simulink model "MiniHelicopterControl"  (R2022b)
settings: Solver=FixedStepAuto  StartTime=0.0  StopTime=30  FixedStep=0.001  RelTol=1e-3
libraries: simulink x1
settings Model: PauseTimes=1  Creator=22438  LastModifiedBy=22438

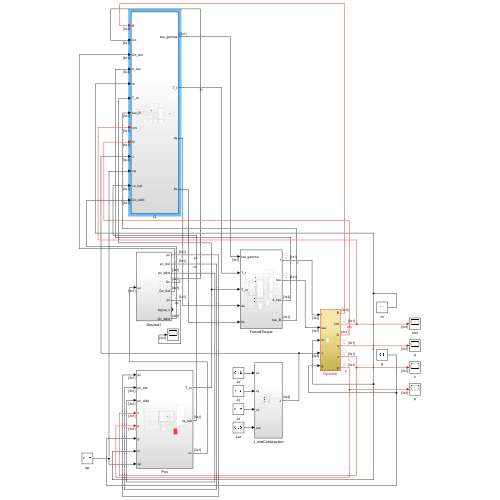
[thumbnail: Simulink's stored preview of the top-level diagram]
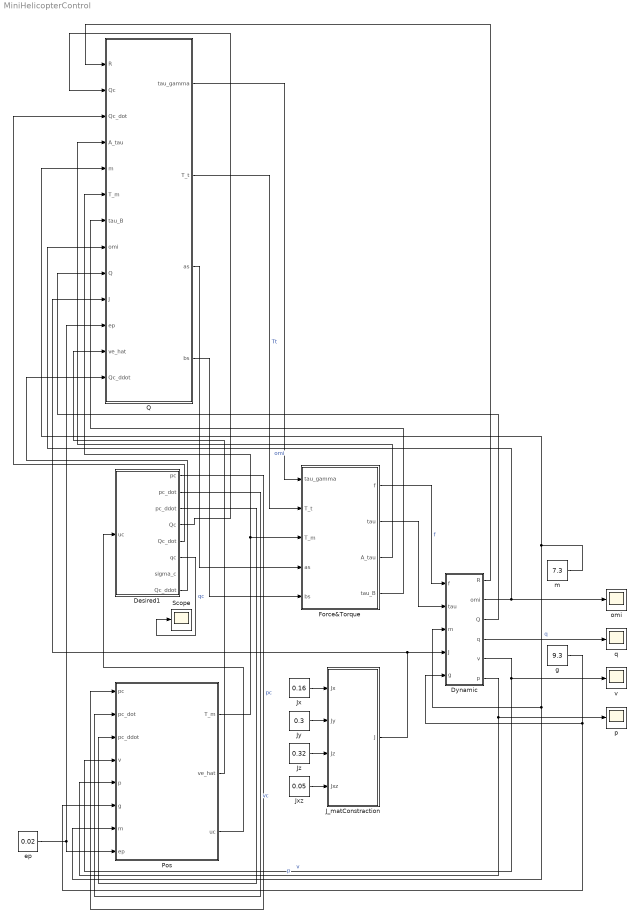
== system MiniHelicopterControl ==
  Desired1 : Subsystem
  Dynamic : Subsystem
  Force&Torque : Subsystem
  J_matConstraction : Subsystem
  Jx : Constant  Value=0.16
  Jxz : Constant  Value=0.05
  Jy : Constant  Value=0.3
  Jz : Constant  Value=0.32
  Pos : Subsystem
  Q : Subsystem
  Scope : Scope
  ep : Constant  Value=0.02
  g : Constant  Value=9.3
  m : Constant  Value=7.3
  omi : Scope
  p : Scope
  q : Scope
  v : Scope
  wires:
  J_matConstraction/1(J) -> Dynamic/4(J), Q/10(J)
  Desired1/1(pc) -> Pos/1(pc)  "pc"
  Desired1/2(pc_dot) -> Pos/2(pc_dot)  "vc"
  Desired1/3(pc_ddot) -> Pos/3(pc_ddot)
  Pos/1(T_m) -> Q/6(T_m), Force&Torque/3(T_m)
  Desired1/4(Qc) -> Q/2(Qc)
  Desired1/5(Qc_dot) -> Q/3(Qc_dot)
  Force&Torque/3(A_tau) -> Q/4(A_tau)
  Force&Torque/4(tau_B) -> Q/7(tau_B)
  ep/1 -> Pos/8(ep), Q/11(ep)
  Pos/2(ve_hat) -> Q/12(ve_hat)
  Q/1(tau_gamma) -> Force&Torque/1(tau_gamma)
  Q/2(T_t) -> Force&Torque/2(T_t)  "Tt"
  Jxz/1 -> J_matConstraction/4(Jxz)
  Jx/1 -> J_matConstraction/1(Jx)
  Jz/1 -> J_matConstraction/3(Jz)
  Jy/1 -> J_matConstraction/2(Jy)
  Q/3(as) -> Force&Torque/4(as)
  Q/4(bs) -> Force&Torque/5(bs)
  m/1 -> Q/5(m), Pos/7(m), Dynamic/3(m)
  Force&Torque/1(f) -> Dynamic/1(f)  "f"
  Force&Torque/2(tau) -> Dynamic/2(tau)
  Dynamic/1(R) -> Q/1(R)
  Dynamic/3(Q) -> Q/9(Q)
  Dynamic/4(q) -> q/1  "q"
  Dynamic/5(v) -> v/1, Pos/4(v)  "v"
  Dynamic/6(p) -> p/1, Pos/5(p)  "p"
  g/1 -> Dynamic/5(g), Pos/6(g)
  Dynamic/2(omi) -> omi/1, Q/8(omi)  "omi"
  Desired1/8(Qc_ddot) -> Q/13(Qc_ddot)
  Pos/3(uc) -> Desired1/1(uc)
  Desired1/6(qc) -> Scope/1  "qc"

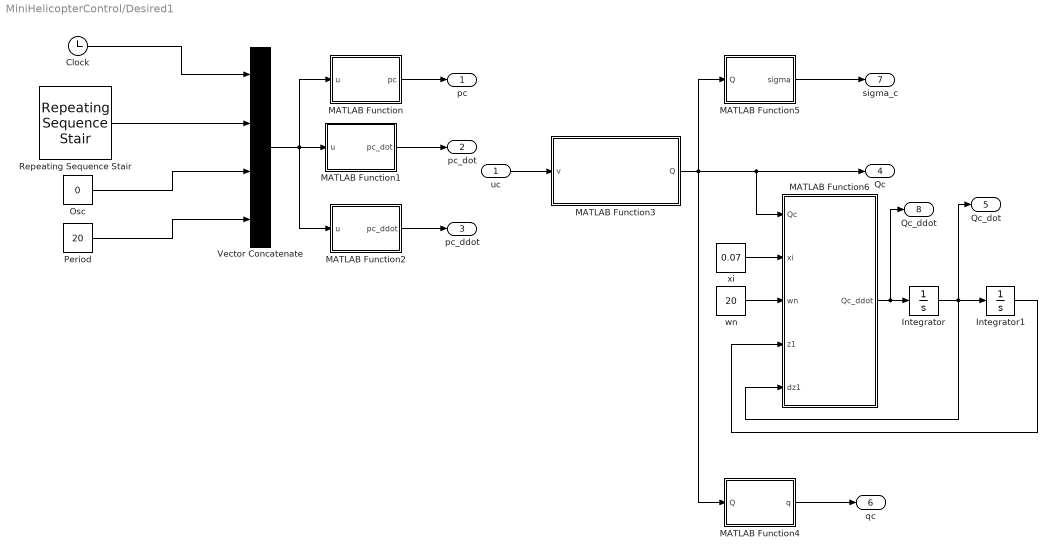
== system MiniHelicopterControl/Desired1 ==
  uc : Inport
  Clock : Clock
  Integrator : Integrator
  Integrator1 : Integrator
  MATLAB Function : MATLAB Function  TreatAsAtomicUnit=on
  MATLAB Function1 : MATLAB Function  TreatAsAtomicUnit=on
  MATLAB Function2 : MATLAB Function  TreatAsAtomicUnit=on
  MATLAB Function3 : MATLAB Function  TreatAsAtomicUnit=on
  MATLAB Function4 : MATLAB Function  TreatAsAtomicUnit=on
  MATLAB Function5 : MATLAB Function  TreatAsAtomicUnit=on
  MATLAB Function6 : MATLAB Function  TreatAsAtomicUnit=on
  Osc : Constant  Value=0
  Period : Constant  Value=20
  Repeating Sequence Stair : simulink/Sources/Repeating Sequence Stair  OutValues=[3].'  tsamp=-1  OutMin=[]  OutMax=[]  OutDataTypeStr=double  OutputDataTypeScalingMode=double  OutDataType=fixdt(0,8)  ConRadixGroup=Best Precision: Vector-wise  OutScaling=2^-12
  Vector Concatenate : Concatenate  NumInputs=4
  wn : Constant  Value=20
  xi : Constant  Value=0.07
  pc : Outport
  pc_dot : Outport  Port=2
  pc_ddot : Outport  Port=3
  Qc : Outport  Port=4
  Qc_dot : Outport  Port=5
  qc : Outport  Port=6
  sigma_c : Outport  Port=7
  Qc_ddot : Outport  Port=8
  wires:
  Repeating Sequence Stair/1 -> Vector Concatenate/2
  Period/1 -> Vector Concatenate/4
  Clock/1 -> Vector Concatenate/1
  MATLAB Function/1(pc) -> pc/1
  Osc/1 -> Vector Concatenate/3
  Vector Concatenate/1 -> MATLAB Function2/1(u), MATLAB Function1/1(u), MATLAB Function/1(u)
  MATLAB Function1/1(pc_dot) -> pc_dot/1
  MATLAB Function2/1(pc_ddot) -> pc_ddot/1
  MATLAB Function4/1(q) -> qc/1
  MATLAB Function5/1(sigma) -> sigma_c/1
  MATLAB Function3/1(Q) -> MATLAB Function4/1(Q), MATLAB Function5/1(Q), Qc/1, MATLAB Function6/1(Qc)
  xi/1 -> MATLAB Function6/2(xi)
  wn/1 -> MATLAB Function6/3(wn)
  MATLAB Function6/1(Qc_ddot) -> Qc_ddot/1, Integrator/1
  Integrator/1 -> Qc_dot/1, MATLAB Function6/5(dz1), Integrator1/1
  Integrator1/1 -> MATLAB Function6/4(z1)
  uc/1 -> MATLAB Function3/1(v)

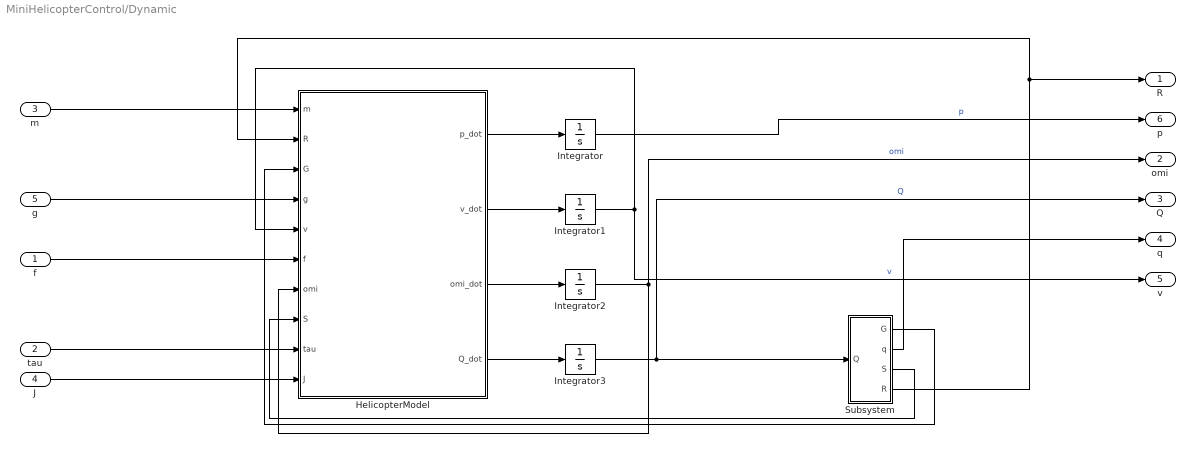
== system MiniHelicopterControl/Dynamic ==
  f : Inport
  tau : Inport  Port=2
  m : Inport  Port=3
  J : Inport  Port=4
  g : Inport  Port=5
  HelicopterModel : MATLAB Function  TreatAsAtomicUnit=on
  Integrator : Integrator  InitialCondition=[1;1;0]
  Integrator1 : Integrator
  Integrator2 : Integrator
  Integrator3 : Integrator  InitialCondition=[sqrt(3)/2;1/2;0;0]
  Subsystem : Subsystem
  R : Outport
  omi : Outport  Port=2
  Q : Outport  Port=3
  q : Outport  Port=4
  v : Outport  Port=5
  p : Outport  Port=6
  wires:
  Integrator1/1 -> v/1, HelicopterModel/5(v)  "v"
  Integrator3/1 -> Subsystem/1(Q), Q/1  "Q"
  Integrator2/1 -> omi/1, HelicopterModel/7(omi)  "omi"
  HelicopterModel/4(Q_dot) -> Integrator3/1
  Integrator/1 -> p/1  "p"
  HelicopterModel/3(omi_dot) -> Integrator2/1
  HelicopterModel/1(p_dot) -> Integrator/1
  J/1 -> HelicopterModel/10(J)
  HelicopterModel/2(v_dot) -> Integrator1/1
  g/1 -> HelicopterModel/4(g)
  tau/1 -> HelicopterModel/9(tau)
  f/1 -> HelicopterModel/6(f)
  m/1 -> HelicopterModel/1(m)
  Subsystem/4(R) -> HelicopterModel/2(R), R/1
  Subsystem/1(G) -> HelicopterModel/3(G)
  Subsystem/2(q) -> q/1
  Subsystem/3(S) -> HelicopterModel/8(S)

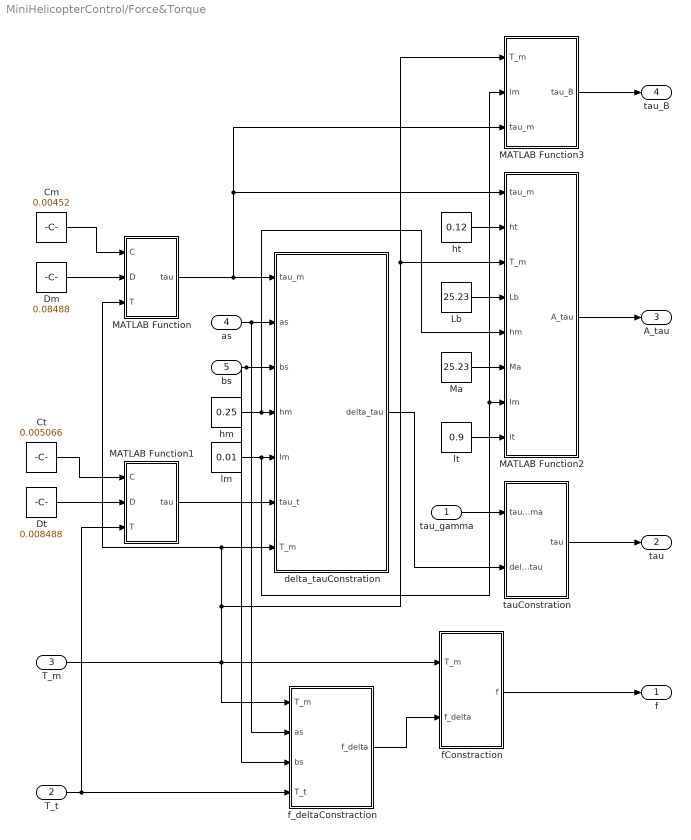
== system MiniHelicopterControl/Force&Torque ==
  tau_gamma : Inport
  T_t : Inport  Port=2
  T_m : Inport  Port=3
  as : Inport  Port=4
  bs : Inport  Port=5
  Cm : Constant  Value=0.00452
  Ct : Constant  Value=0.005066
  Dm : Constant  Value=0.08488
  Dt : Constant  Value=0.008488
  Lb : Constant  Value=25.23
  MATLAB Function : MATLAB Function  TreatAsAtomicUnit=on
  MATLAB Function1 : MATLAB Function  TreatAsAtomicUnit=on
  MATLAB Function2 : MATLAB Function  TreatAsAtomicUnit=on
  MATLAB Function3 : MATLAB Function  TreatAsAtomicUnit=on
  Ma : Constant  Value=25.23
  delta_tauConstration : MATLAB Function  TreatAsAtomicUnit=on
  fConstraction : MATLAB Function  TreatAsAtomicUnit=on
  f_deltaConstraction : MATLAB Function  TreatAsAtomicUnit=on
  hm : Constant  Value=0.25
  ht : Constant  Value=0.12
  lm : Constant  Value=0.01
  lt : Constant  Value=0.9
  tauConstration : MATLAB Function  TreatAsAtomicUnit=on
  f : Outport
  tau : Outport  Port=2
  A_tau : Outport  Port=3
  tau_B : Outport  Port=4
  wires:
  as/1 -> f_deltaConstraction/2(as), delta_tauConstration/2(as)
  delta_tauConstration/1(delta_tau) -> tauConstration/2(delta_tau)
  lm/1 -> MATLAB Function3/2(lm), MATLAB Function2/7(lm), delta_tauConstration/5(lm)
  T_m/1 -> f_deltaConstraction/1(T_m), fConstraction/1(T_m), MATLAB Function3/1(T_m), MATLAB Function2/3(T_m), MATLAB Function/3(T), delta_tauConstration/7(T_m)
  bs/1 -> delta_tauConstration/3(bs), f_deltaConstraction/3(bs)
  f_deltaConstraction/1(f_delta) -> fConstraction/2(f_delta)
  hm/1 -> MATLAB Function2/5(hm), delta_tauConstration/4(hm)
  T_t/1 -> MATLAB Function1/3(T), f_deltaConstraction/4(T_t)
  MATLAB Function1/1(tau) -> delta_tauConstration/6(tau_t)
  tau_gamma/1 -> tauConstration/1(tau_gamma)
  fConstraction/1(f) -> f/1
  tauConstration/1(tau) -> tau/1
  MATLAB Function/1(tau) -> MATLAB Function3/3(tau_m), MATLAB Function2/1(tau_m), delta_tauConstration/1(tau_m)
  Cm/1 -> MATLAB Function/1(C)
  Dm/1 -> MATLAB Function/2(D)
  Ct/1 -> MATLAB Function1/1(C)
  Dt/1 -> MATLAB Function1/2(D)
  ht/1 -> MATLAB Function2/2(ht)
  Lb/1 -> MATLAB Function2/4(Lb)
  Ma/1 -> MATLAB Function2/6(Ma)
  lt/1 -> MATLAB Function2/8(lt)
  MATLAB Function2/1(A_tau) -> A_tau/1
  MATLAB Function3/1(tau_B) -> tau_B/1

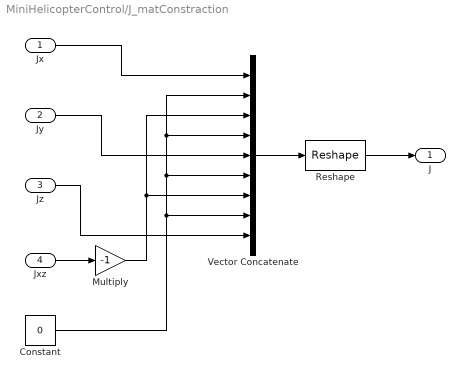
== system MiniHelicopterControl/J_matConstraction ==
  Jx : Inport
  Jy : Inport  Port=2
  Jz : Inport  Port=3
  Jxz : Inport  Port=4
  Constant : Constant  Value=0
  Multiply : Gain  Gain=-1
  Reshape : Reshape  OutputDimensionality=Customize  OutputDimensions=[3,3]
  Vector Concatenate : Concatenate  NumInputs=9
  J : Outport
  wires:
  Jy/1 -> Vector Concatenate/5
  Vector Concatenate/1 -> Reshape/1
  Constant/1 -> Vector Concatenate/8, Vector Concatenate/6, Vector Concatenate/4, Vector Concatenate/2
  Jz/1 -> Vector Concatenate/9
  Jx/1 -> Vector Concatenate/1
  Reshape/1 -> J/1
  Multiply/1 -> Vector Concatenate/7, Vector Concatenate/3
  Jxz/1 -> Multiply/1

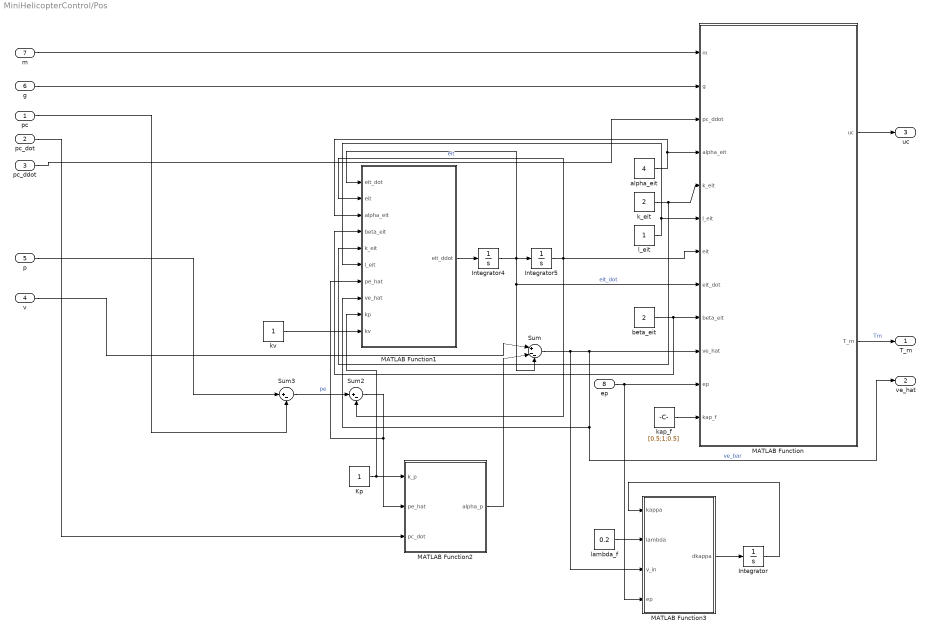
== system MiniHelicopterControl/Pos ==
  pc : Inport
  pc_dot : Inport  Port=2
  pc_ddot : Inport  Port=3
  v : Inport  Port=4
  p : Inport  Port=5
  g : Inport  Port=6
  m : Inport  Port=7
  ep : Inport  Port=8
  Integrator : Integrator
  Integrator4 : Integrator
  Integrator5 : Integrator  InitialCondition=[0.3;0.3;0.3]
  Kp : Constant
  MATLAB Function : MATLAB Function  TreatAsAtomicUnit=on
  MATLAB Function1 : MATLAB Function  TreatAsAtomicUnit=on
  MATLAB Function2 : MATLAB Function  TreatAsAtomicUnit=on
  MATLAB Function3 : MATLAB Function  TreatAsAtomicUnit=on
  Sum : Sum  Inputs=|+--
  Sum2 : Sum  Inputs=|+-
  Sum3 : Sum  Inputs=|+-
  alpha_eit : Constant  Value=4
  beta_eit : Constant  Value=2
  k_eit : Constant  Value=2
  kap_f : Constant  Value=[0.5;1;0.5]
  kv : Constant
  l_eit : Constant
  lambda_f : Constant  Value=0.2
  T_m : Outport
  ve_hat : Outport  Port=2
  uc : Outport  Port=3
  wires:
  k_eit/1 -> MATLAB Function1/5(k_eit), MATLAB Function/5(k_eit)
  beta_eit/1 -> MATLAB Function1/4(beta_eit), MATLAB Function/9(beta_eit)
  Integrator5/1 -> Sum2/2, MATLAB Function/7(eit), MATLAB Function1/2(eit)  "eit"
  l_eit/1 -> MATLAB Function1/6(l_eit), MATLAB Function/6(l_eit)
  Integrator4/1 -> Integrator5/1, MATLAB Function/8(eit_dot), Sum/3, MATLAB Function1/1(eit_dot)  "eit_dot"
  Sum2/1 -> MATLAB Function1/7(pe_hat), MATLAB Function2/2(pe_hat)
  alpha_eit/1 -> MATLAB Function1/3(alpha_eit), MATLAB Function/4(alpha_eit)
  MATLAB Function/2(T_m) -> T_m/1  "Tm"
  MATLAB Function1/1(eit_ddot) -> Integrator4/1
  Integrator/1 -> MATLAB Function3/1(kappa)
  MATLAB Function2/1(alpha_p) -> Sum/2
  v/1 -> Sum/1
  ep/1 -> MATLAB Function3/4(ep), MATLAB Function/11(ep)
  p/1 -> Sum3/1
  Sum3/1 -> Sum2/1  "pe"
  pc_dot/1 -> MATLAB Function2/3(pc_dot)
  pc_ddot/1 -> MATLAB Function/3(pc_ddot)
  pc/1 -> Sum3/2
  g/1 -> MATLAB Function/2(g)
  m/1 -> MATLAB Function/1(m)
  Kp/1 -> MATLAB Function1/9(kp), MATLAB Function2/1(k_p)
  kv/1 -> MATLAB Function1/10(kv)
  MATLAB Function/1(uc) -> uc/1
  MATLAB Function3/1(dkappa) -> Integrator/1
  lambda_f/1 -> MATLAB Function3/2(lambda)
  Sum/1 -> MATLAB Function3/3(v_in), MATLAB Function1/8(ve_hat), ve_hat/1, MATLAB Function/10(ve_hat)  "ve_bar"
  kap_f/1 -> MATLAB Function/12(kap_f)

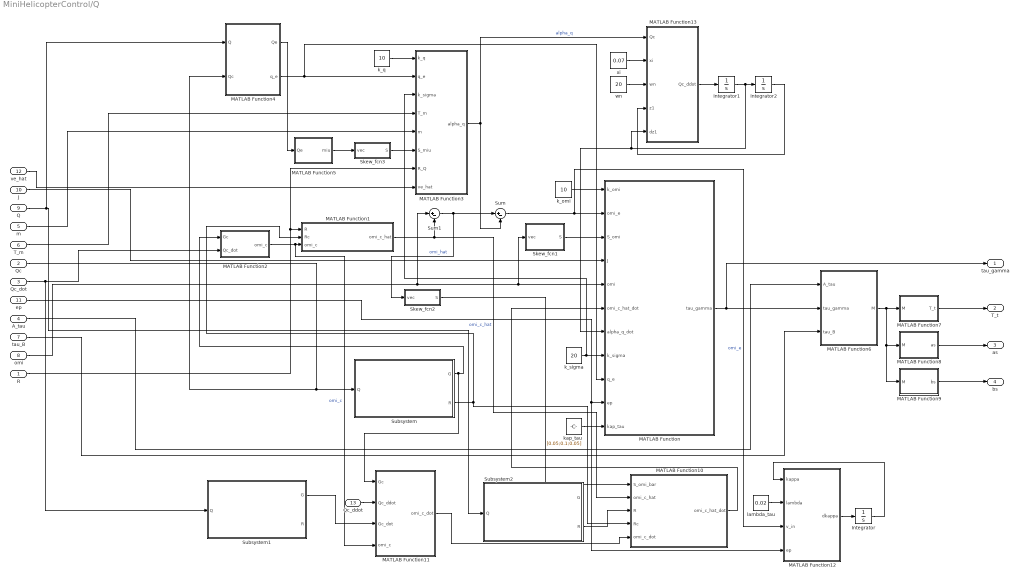
== system MiniHelicopterControl/Q ==
  R : Inport
  Qc : Inport  Port=2
  Qc_dot : Inport  Port=3
  A_tau : Inport  Port=4
  m : Inport  Port=5
  T_m : Inport  Port=6
  tau_B : Inport  Port=7
  omi : Inport  Port=8
  Q : Inport  Port=9
  J : Inport  Port=10
  ep : Inport  Port=11
  ve_hat : Inport  Port=12
  Qc_ddot : Inport  Port=13
  Integrator : Integrator
  Integrator1 : Integrator
  Integrator2 : Integrator
  MATLAB Function : MATLAB Function  TreatAsAtomicUnit=on
  MATLAB Function1 : MATLAB Function  TreatAsAtomicUnit=on
  MATLAB Function10 : MATLAB Function  TreatAsAtomicUnit=on
  MATLAB Function11 : MATLAB Function  TreatAsAtomicUnit=on
  MATLAB Function12 : MATLAB Function  TreatAsAtomicUnit=on
  MATLAB Function13 : MATLAB Function  TreatAsAtomicUnit=on
  MATLAB Function2 : MATLAB Function  TreatAsAtomicUnit=on
  MATLAB Function3 : MATLAB Function  TreatAsAtomicUnit=on
  MATLAB Function4 : MATLAB Function  TreatAsAtomicUnit=on
  MATLAB Function5 : MATLAB Function  TreatAsAtomicUnit=on
  MATLAB Function6 : MATLAB Function  TreatAsAtomicUnit=on
  MATLAB Function7 : MATLAB Function  TreatAsAtomicUnit=on
  MATLAB Function8 : MATLAB Function  TreatAsAtomicUnit=on
  MATLAB Function9 : MATLAB Function  TreatAsAtomicUnit=on
  Skew_fcn1 : MATLAB Function  TreatAsAtomicUnit=on
  Skew_fcn2 : MATLAB Function  TreatAsAtomicUnit=on
  Skew_fcn3 : MATLAB Function  TreatAsAtomicUnit=on
  Subsystem : Subsystem
  Subsystem1 : Subsystem
  Subsystem2 : Subsystem
  Sum : Sum  Inputs=|+-
  Sum1 : Sum  Inputs=|+-
  k_omi : Constant  Value=10
  k_q : Constant  Value=10
  k_sigma : Constant  Value=20
  kap_tau : Constant  Value=[0.05;0.1;0.05]
  lambda_tau : Constant  Value=0.02
  wn : Constant  Value=20
  xi : Constant  Value=0.07
  tau_gamma : Outport
  T_t : Outport  Port=2
  as : Outport  Port=3
  bs : Outport  Port=4
  wires:
  T_m/1 -> MATLAB Function3/4(T_m)
  A_tau/1 -> MATLAB Function6/1(A_tau)
  Integrator/1 -> MATLAB Function12/1(kappa)
  MATLAB Function3/1(alpha_q) -> MATLAB Function13/1(Qc), Sum/2  "alpha_q"
  MATLAB Function/1(tau_gamma) -> tau_gamma/1, MATLAB Function6/2(tau_gamma)
  k_q/1 -> MATLAB Function3/1(k_q)
  k_sigma/1 -> MATLAB Function3/3(k_sigma), MATLAB Function/8(k_sigma)
  Qc/1 -> Subsystem/1(Q), MATLAB Function4/2(Qc)
  MATLAB Function4/2(q_e) -> MATLAB Function/9(q_e), MATLAB Function3/2(q_e)
  ep/1 -> MATLAB Function12/4(ep), MATLAB Function/10(ep)
  Q/1 -> Subsystem2/1(Q), MATLAB Function4/1(Q)
  omi/1 -> Skew_fcn1/1(vec), MATLAB Function/5(omi), Sum1/1
  MATLAB Function6/1(M) -> MATLAB Function9/1(M), MATLAB Function8/1(M), MATLAB Function7/1(M)
  MATLAB Function1/1(omi_c_hat) -> MATLAB Function10/2(omi_c_hat), Sum1/2  "omi_c_hat"
  MATLAB Function4/1(Qe) -> MATLAB Function5/1(Qe)
  Sum/1 -> MATLAB Function12/3(v_in), MATLAB Function/2(omi_e)  "omi_e"
  Skew_fcn1/1(S) -> MATLAB Function/3(S_omi)
  Integrator1/1 -> MATLAB Function/7(alpha_q_dot), MATLAB Function13/5(dz1), Integrator2/1
  Sum1/1 -> Skew_fcn2/1(vec), Sum/1  "omi_hat"
  ve_hat/1 -> MATLAB Function3/8(ve_hat)
  MATLAB Function5/1(miu) -> Skew_fcn3/1(vec)
  Skew_fcn3/1(S) -> MATLAB Function3/6(S_miu)
  R/1 -> MATLAB Function3/7(R_Q), MATLAB Function1/1(R)
  MATLAB Function2/1(omi_c) -> MATLAB Function11/4(omi_c), MATLAB Function1/3(omi_c)  "omi_c"
  J/1 -> MATLAB Function/4(J)
  k_omi/1 -> MATLAB Function/1(k_omi)
  m/1 -> MATLAB Function3/5(m)
  Qc_dot/1 -> Subsystem1/1(Q), MATLAB Function2/2(Qc_dot)
  tau_B/1 -> MATLAB Function6/3(tau_B)
  MATLAB Function7/1(T_t) -> T_t/1
  MATLAB Function8/1(as) -> as/1
  MATLAB Function9/1(bs) -> bs/1
  Subsystem/1(G) -> MATLAB Function11/1(Gc), MATLAB Function2/1(Gc)
  Subsystem/2(R) -> MATLAB Function1/2(Rc), MATLAB Function10/4(Rc)
  MATLAB Function10/1(omi_c_hat_dot) -> MATLAB Function/6(omi_c_hat_dot)
  Skew_fcn2/1(S) -> MATLAB Function10/1(S_omi_bar)
  Subsystem1/1(G) -> MATLAB Function11/3(Gc_dot)
  Qc_ddot/1 -> MATLAB Function11/2(Qc_ddot)
  MATLAB Function11/1(omi_c_dot) -> MATLAB Function10/5(omi_c_dot)
  Subsystem2/2(R) -> MATLAB Function10/3(R)
  MATLAB Function12/1(dkappa) -> Integrator/1
  lambda_tau/1 -> MATLAB Function12/2(lambda)
  kap_tau/1 -> MATLAB Function/11(kap_tau)
  xi/1 -> MATLAB Function13/2(xi)
  wn/1 -> MATLAB Function13/3(wn)
  MATLAB Function13/1(Qc_ddot) -> Integrator1/1
  Integrator2/1 -> MATLAB Function13/4(z1)

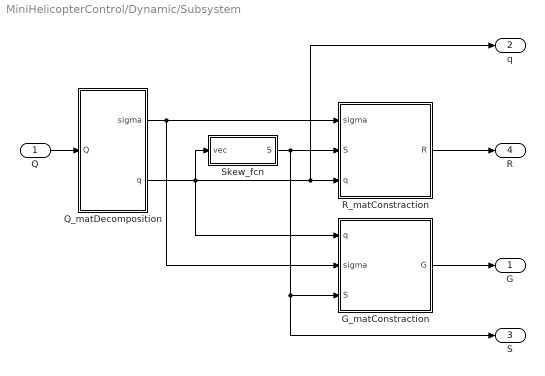
== system MiniHelicopterControl/Dynamic/Subsystem ==
  Q : Inport
  G_matConstraction : MATLAB Function  TreatAsAtomicUnit=on
  Q_matDecomposition : MATLAB Function  TreatAsAtomicUnit=on
  R_matConstraction : MATLAB Function  TreatAsAtomicUnit=on
  Skew_fcn : MATLAB Function  TreatAsAtomicUnit=on
  G : Outport
  q : Outport  Port=2
  S : Outport  Port=3
  R : Outport  Port=4
  wires:
  Q/1 -> Q_matDecomposition/1(Q)
  Q_matDecomposition/2(q) -> Skew_fcn/1(vec), q/1, R_matConstraction/3(q), G_matConstraction/1(q)
  R_matConstraction/1(R) -> R/1
  Skew_fcn/1(S) -> S/1, G_matConstraction/3(S), R_matConstraction/2(S)
  Q_matDecomposition/1(sigma) -> G_matConstraction/2(sigma), R_matConstraction/1(sigma)
  G_matConstraction/1(G) -> G/1

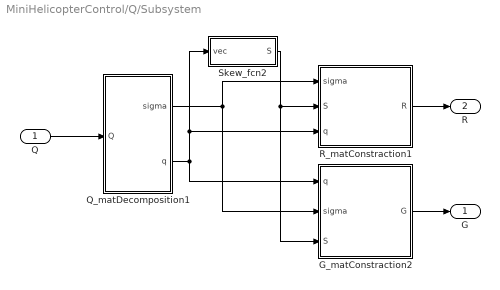
== system MiniHelicopterControl/Q/Subsystem ==
  Q : Inport
  G_matConstraction2 : MATLAB Function  TreatAsAtomicUnit=on
  Q_matDecomposition1 : MATLAB Function  TreatAsAtomicUnit=on
  R_matConstraction1 : MATLAB Function  TreatAsAtomicUnit=on
  Skew_fcn2 : MATLAB Function  TreatAsAtomicUnit=on
  G : Outport
  R : Outport  Port=2
  wires:
  Q_matDecomposition1/2(q) -> Skew_fcn2/1(vec), R_matConstraction1/3(q), G_matConstraction2/1(q)
  R_matConstraction1/1(R) -> R/1
  Skew_fcn2/1(S) -> G_matConstraction2/3(S), R_matConstraction1/2(S)
  Q_matDecomposition1/1(sigma) -> R_matConstraction1/1(sigma), G_matConstraction2/2(sigma)
  G_matConstraction2/1(G) -> G/1
  Q/1 -> Q_matDecomposition1/1(Q)

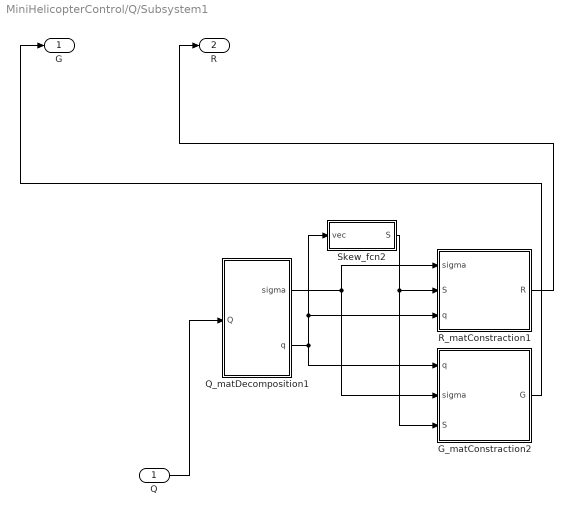
== system MiniHelicopterControl/Q/Subsystem1 ==
  Q : Inport
  G_matConstraction2 : MATLAB Function  TreatAsAtomicUnit=on
  Q_matDecomposition1 : MATLAB Function  TreatAsAtomicUnit=on
  R_matConstraction1 : MATLAB Function  TreatAsAtomicUnit=on
  Skew_fcn2 : MATLAB Function  TreatAsAtomicUnit=on
  G : Outport
  R : Outport  Port=2
  wires:
  Q_matDecomposition1/2(q) -> Skew_fcn2/1(vec), R_matConstraction1/3(q), G_matConstraction2/1(q)
  R_matConstraction1/1(R) -> R/1
  Skew_fcn2/1(S) -> G_matConstraction2/3(S), R_matConstraction1/2(S)
  Q_matDecomposition1/1(sigma) -> R_matConstraction1/1(sigma), G_matConstraction2/2(sigma)
  G_matConstraction2/1(G) -> G/1
  Q/1 -> Q_matDecomposition1/1(Q)

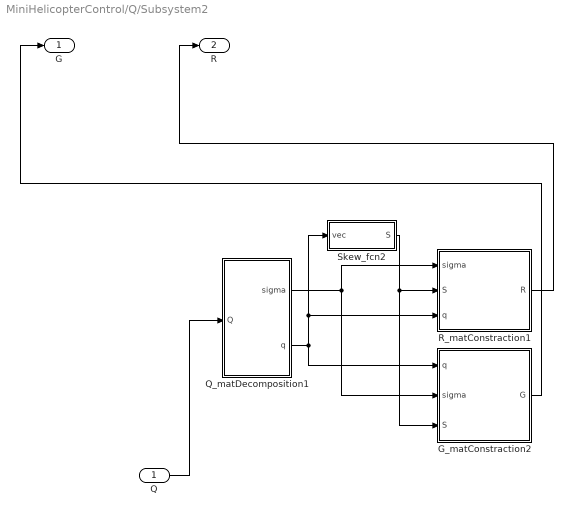
== system MiniHelicopterControl/Q/Subsystem2 ==
  Q : Inport
  G_matConstraction2 : MATLAB Function  TreatAsAtomicUnit=on
  Q_matDecomposition1 : MATLAB Function  TreatAsAtomicUnit=on
  R_matConstraction1 : MATLAB Function  TreatAsAtomicUnit=on
  Skew_fcn2 : MATLAB Function  TreatAsAtomicUnit=on
  G : Outport
  R : Outport  Port=2
  wires:
  Q_matDecomposition1/2(q) -> Skew_fcn2/1(vec), R_matConstraction1/3(q), G_matConstraction2/1(q)
  R_matConstraction1/1(R) -> R/1
  Skew_fcn2/1(S) -> G_matConstraction2/3(S), R_matConstraction1/2(S)
  Q_matDecomposition1/1(sigma) -> R_matConstraction1/1(sigma), G_matConstraction2/2(sigma)
  G_matConstraction2/1(G) -> G/1
  Q/1 -> Q_matDecomposition1/1(Q)

== matlab function MiniHelicopterControl/Q/MATLAB Function10 ==
  data: omi_c_hat_dot output; S_omi_bar input; omi_c_hat input; R input; Rc input; omi_c_dot input
function omi_c_hat_dot = fcn(S_omi_bar, omi_c_hat, R, Rc, omi_c_dot)
omi_c_hat_dot = -S_omi_bar*omi_c_hat + R*Rc'*omi_c_dot;
end

== matlab function MiniHelicopterControl/Q/Skew_fcn2 ==
  data: vec input; S output
function S = fcn(vec)
v = vec;
vx = v(1);
vy = v(2);
vz = v(3);

S = [ ...
    0, -vz, vy; ...
    vz, 0, -vx; ...
    -vy, vx, 0 ...
    ];
end

== matlab function MiniHelicopterControl/Q/MATLAB Function11 ==
  data: Gc input; omi_c_dot output; Qc_ddot input; Gc_dot input; omi_c input
function omi_c_dot = fcn(Gc, Qc_ddot, Gc_dot, omi_c)
omi_c_dot = Gc'*(Qc_ddot - Gc_dot*omi_c);
end

== matlab function MiniHelicopterControl/Pos/MATLAB Function ==
  data: uc output size=[3 1]; m input; g input; T_m output size=1; pc_ddot input; alpha_eit input; k_eit input; l_eit input; eit input; eit_dot input; beta_eit input; ve_hat input; ep input; kap_f input
function [uc,T_m]= fcn(m, g, pc_ddot, alpha_eit, k_eit, l_eit, eit, eit_dot, beta_eit, ve_hat, ep, kap_f)
uc = g.*[0;0;1] + pc_ddot - alpha_eit.*tanh(k_eit.*eit + l_eit.*eit_dot) - ...
    beta_eit.*tanh(l_eit.*eit_dot) - tanh(diag(ve_hat./ep))*kap_f;
T_m = m*norm(uc);
end

== matlab function MiniHelicopterControl/Pos/MATLAB Function3 ==
  data: kappa input; dkappa output; lambda input; v_in input; ep input
function dkappa = fcn(kappa, lambda, v_in, ep)
dkappa = lambda*tanh(v_in/ep).*v_in-0.002*kappa;
end

== matlab function MiniHelicopterControl/Q/Subsystem1/G_matConstraction2 ==
  data: q input; sigma input; G output; S input
function G = fcn(q, sigma, S)
G = 0.5.*[-1.*q';...
    sigma.*eye(3) + S];
end

== matlab function MiniHelicopterControl/Q/Subsystem1/Q_matDecomposition1 ==
  data: Q input; sigma output; q output
function [sigma, q] = fcn(Q)
sigma = Q(1);
q = [Q(2);Q(3);Q(4)];
end

== matlab function MiniHelicopterControl/Q/MATLAB Function12 ==
  data: kappa input; dkappa output; lambda input; v_in input; ep input
function dkappa = fcn(kappa, lambda, v_in, ep)
dkappa = lambda*tanh(v_in/ep).*v_in-0.002*kappa;
end

== matlab function MiniHelicopterControl/Q/Subsystem1/R_matConstraction1 ==
  data: sigma input; R output; S input; q input
function R = fcn(sigma, S, q)
R = (sigma^2 - q'*q)*eye(3) + 2*q*q' - 2*sigma*S;
end

== matlab function MiniHelicopterControl/Dynamic/Subsystem/Q_matDecomposition ==
  data: Q input; sigma output; q output
function [sigma, q] = fcn(Q)
sigma = Q(1);
q = [Q(2);Q(3);Q(4)];
end

== matlab function MiniHelicopterControl/Pos/MATLAB Function1 ==
  data: eit_dot input; eit_ddot output; eit input; alpha_eit input; beta_eit input; k_eit input; l_eit input; pe_hat input; ve_hat input; kp input; kv input
function eit_ddot = fcn(eit_dot, eit, alpha_eit, beta_eit, k_eit, l_eit, pe_hat, ve_hat, kp, kv)
eit_ddot = -alpha_eit.*tanh(k_eit.*eit + l_eit.*eit_dot) - beta_eit.*tanh(l_eit.*eit_dot) - (kp^2-1)*pe_hat + (kv+kp)*ve_hat;
end

== matlab function MiniHelicopterControl/Pos/MATLAB Function2 ==
  data: k_p input; alpha_p output; pe_hat input; pc_dot input
function alpha_p = fcn(k_p, pe_hat, pc_dot)
alpha_p = -k_p.*pe_hat + pc_dot;
end

== matlab function MiniHelicopterControl/Force&Torque/MATLAB Function ==
  data: C input; tau output; D input; T input
function tau = fcn(C, D, T)
tau = C*abs(T)^1.5 + D;
end

== matlab function MiniHelicopterControl/Force&Torque/MATLAB Function1 ==
  data: C input; tau output; D input; T input
function tau = fcn(C, D, T)
tau = C*abs(T)^1.5 + D;
end

== matlab function MiniHelicopterControl/Q/MATLAB Function ==
  data: k_omi input; tau_gamma output size=[3 1]; omi_e input; S_omi input; J input; omi input; omi_c_hat_dot input; alpha_q_dot input; k_sigma input; q_e input; ep input; kap_tau input
function tau_gamma = fcn(k_omi, omi_e, S_omi, J, omi, omi_c_hat_dot, alpha_q_dot, k_sigma, q_e, ep, kap_tau)
tau_gamma = -k_omi*omi_e + S_omi*J*omi + J*(omi_c_hat_dot+alpha_q_dot) - k_sigma*q_e - tanh(diag(omi_e./ep))*kap_tau;
end

== matlab function MiniHelicopterControl/Q/Skew_fcn1 ==
  data: vec input; S output
function S = fcn(vec)
v = vec;
vx = v(1);
vy = v(2);
vz = v(3);

S = [ ...
    0, -vz, vy; ...
    vz, 0, -vx; ...
    -vy, vx, 0 ...
    ];
end

== matlab function MiniHelicopterControl/Q/MATLAB Function1 ==
  data: R input; omi_c_hat output; Rc input; omi_c input
function omi_c_hat = fcn(R, Rc, omi_c)
omi_c_hat = R*Rc'*omi_c;
end

== matlab function MiniHelicopterControl/Dynamic/HelicopterModel ==
  data: m input; p_dot output size=[3 1]; R input; G input; g input; v input; f input; omi input; S input; tau input; J input; v_dot output size=[3 1]; omi_dot output size=[3 1]; Q_dot output size=[4 1]
function [p_dot, v_dot, omi_dot, Q_dot] = fcn(m, R, G, g, v, f, omi, S, tau, J)
p_dot = v;
v_dot = -g.*[0; 0; 1] + 1/m*R'*f;
Q_dot = G*omi;
omi_dot = J^(-1)*(-1*S*J*omi + tau);
end

== matlab function MiniHelicopterControl/Q/Subsystem/Q_matDecomposition1 ==
  data: Q input; sigma output; q output
function [sigma, q] = fcn(Q)
sigma = Q(1);
q = [Q(2);Q(3);Q(4)];
end

== matlab function MiniHelicopterControl/Q/Subsystem/R_matConstraction1 ==
  data: sigma input; R output; S input; q input
function R = fcn(sigma, S, q)
R = (sigma^2 - q'*q)*eye(3) + 2*(q*q') - 2*sigma*S;
end

== matlab function MiniHelicopterControl/Q/Subsystem/Skew_fcn2 ==
  data: vec input; S output
function S = fcn(vec)
v = vec;
vx = v(1);
vy = v(2);
vz = v(3);

S = [ ...
    0, -vz, vy; ...
    vz, 0, -vx; ...
    -vy, vx, 0 ...
    ];
end

== matlab function MiniHelicopterControl/Q/Skew_fcn3 ==
  data: vec input; S output
function S = fcn(vec)
v = vec;
vx = v(1);
vy = v(2);
vz = v(3);

S = [ ...
    0, -vz, vy; ...
    vz, 0, -vx; ...
    -vy, vx, 0 ...
    ];
end

== matlab function MiniHelicopterControl/Q/Subsystem/G_matConstraction2 ==
  data: q input; sigma input; G output; S input
function G = fcn(q, sigma, S)
G = 0.5.*[-1.*q';...
    sigma.*eye(3) + S];
end

== matlab function MiniHelicopterControl/Q/MATLAB Function2 ==
  data: Gc input; omi_c output; Qc_dot input
function omi_c = fcn(Gc, Qc_dot)
omi_c = Gc'*Qc_dot;
end

== matlab function MiniHelicopterControl/Q/MATLAB Function3 ==
  data: k_q input; alpha_q output; q_e input; k_sigma input; T_m input; m input; S_miu input; R_Q input; ve_hat input
function alpha_q = fcn(k_q, q_e, k_sigma, T_m, m, S_miu, R_Q, ve_hat)
alpha_q = -k_q.*q_e - 2/k_sigma*T_m/m*S_miu'*R_Q*ve_hat;
end

== matlab function MiniHelicopterControl/Q/MATLAB Function4 ==
  data: Q input; Qe output; Qc input; q_e output
function [Qe,q_e]= fcn(Q, Qc)
Q1 = [Qc(1);Qc(2);Qc(3);Qc(4)];
Q2 = Q;
sigma1 = Q1(1);
q1 = Q1(2:4);
sigma2 = Q2(1);
q2 = Q2(2:4);
v = q1;
vx = v(1);
vy = v(2);
vz = v(3);
S_q1 = [ ...
    0, -vz, vy; ...
    vz, 0, -vx; ...
    -vy, vx, 0 ...
    ];
Qe = [sigma1*sigma2-q1'*q2;
    sigma1.*q2+sigma2.*q1+S_q1*q2];
q_e = Qe(2:4);
end

== matlab function MiniHelicopterControl/Q/MATLAB Function5 ==
  data: Qe input; miu output
function miu = fcn(Qe)

miu = [Qe(3);-Qe(2);-Qe(1)];
end

== matlab function MiniHelicopterControl/Q/MATLAB Function6 ==
  data: A_tau input; M output size=[3 1]; tau_gamma input; tau_B input
function M = fcn(A_tau, tau_gamma, tau_B)
M = A_tau^(-1)*(tau_gamma - tau_B);
end

== matlab function MiniHelicopterControl/Force&Torque/MATLAB Function2 ==
  data: tau_m input; A_tau output; ht input; T_m input; Lb input; hm input; Ma input; lm input; lt input
function A_tau = fcn(tau_m, ht, T_m, Lb, hm, Ma, lm, lt)
A_tau = [ht tau_m T_m*hm+Lb;
    0 T_m*hm+Ma -tau_m;
    -lt 0 -T_m*lm];
end

== matlab function MiniHelicopterControl/Force&Torque/MATLAB Function3 ==
  data: T_m input; tau_B output; lm input; tau_m input
function tau_B = fcn(T_m, lm, tau_m)
tau_B = [0;T_m*lm;tau_m];
end

== matlab function MiniHelicopterControl/Q/MATLAB Function7 ==
  data: M input; T_t output
function T_t = fcn(M)
T_t = M(1);
end

== matlab function MiniHelicopterControl/Q/MATLAB Function8 ==
  data: M input; as output
function as = fcn(M)
as = M(2);
end

== matlab function MiniHelicopterControl/Q/MATLAB Function9 ==
  data: M input; bs output
function bs = fcn(M)
bs = M(3);
end

== matlab function MiniHelicopterControl/Desired1/MATLAB Function ==
  data: u input; pc output
function pc = fcn(u)
pc_x = 5*cos(2*pi/u(4)*u(1));
pc_y = 5*sin(4*pi/u(4)*u(1));
pc_z = 5;
pc = [pc_x;pc_y;pc_z];
end

== matlab function MiniHelicopterControl/Desired1/MATLAB Function1 ==
  data: u input; pc_dot output
function pc_dot = fcn(u)
pc_x_dot = -10*pi/u(4)*sin(2*pi/u(4)*u(1));
pc_y_dot = 20*pi/u(4)*cos(4*pi/u(4)*u(1));
pc_z_dot = 0;
pc_dot = [pc_x_dot;pc_y_dot;pc_z_dot];
end

== matlab function MiniHelicopterControl/Desired1/MATLAB Function2 ==
  data: u input; pc_ddot output
function pc_ddot = fcn(u)
pc_x_ddot = -20*pi^2/(u(4)^2)*cos(2*pi/u(4)*u(1));
pc_y_ddot = -80*pi^2/(u(4)^2)*sin(4*pi/u(4)*u(1));
pc_z_ddot = 0;
pc_ddot = [pc_x_ddot;pc_y_ddot;pc_z_ddot];
end

== matlab function MiniHelicopterControl/Desired1/MATLAB Function3 ==
  data: v input; Q output
function Q = vectorToQuaternion(v)
ucx = v(1);
ucy = v(2);
ucz = v(3);
uc = v;
sigmac = sqrt(1/2+ucz/2/norm(uc));
qc = 1/2/norm(uc)/sigmac*[ucy,-ucx,0]';
Q = [sigmac,qc']';
end

== matlab function MiniHelicopterControl/Desired1/MATLAB Function4 ==
  data: Q input; q output
function q = fcn(Q)
q = [Q(2);Q(3);Q(4)];
end

== matlab function MiniHelicopterControl/Desired1/MATLAB Function5 ==
  data: Q input; sigma output
function sigma = fcn(Q)
sigma = Q(1);
end

== matlab function MiniHelicopterControl/Desired1/MATLAB Function6 ==
  data: Qc input size=[4 1]; Qc_ddot output size=[4 1]; xi input; wn input; z1 input; dz1 input
function Qc_ddot= fcn(Qc,xi,wn,z1,dz1)
ddz1 = -2*xi*wn*dz1-wn*(z1-Qc);
Qc_ddot = ddz1;
end

== matlab function MiniHelicopterControl/Q/Subsystem1/Skew_fcn2 ==
  data: vec input; S output
function S = fcn(vec)
v = vec;
vx = v(1);
vy = v(2);
vz = v(3);

S = [ ...
    0, -vz, vy; ...
    vz, 0, -vx; ...
    -vy, vx, 0 ...
    ];
end

== matlab function MiniHelicopterControl/Dynamic/Subsystem/R_matConstraction ==
  data: sigma input; R output; S input; q input
function R = fcn(sigma, S, q)
R = (sigma^2 - q'*q)*eye(3) + 2*(q*q') - 2.*sigma*S;
end

== matlab function MiniHelicopterControl/Q/Subsystem2/G_matConstraction2 ==
  data: q input; sigma input; G output; S input
function G = fcn(q, sigma, S)
G = 0.5.*[-1.*q';...
    sigma.*eye(3) + S];
end

== matlab function MiniHelicopterControl/Q/Subsystem2/Q_matDecomposition1 ==
  data: Q input; sigma output; q output
function [sigma, q] = fcn(Q)
sigma = Q(1);
q = [Q(2);Q(3);Q(4)];
end

== matlab function MiniHelicopterControl/Q/Subsystem2/R_matConstraction1 ==
  data: sigma input; R output; S input; q input
function R = fcn(sigma, S, q)
R = (sigma^2 - q'*q)*eye(3) + 2*q*q' - 2*sigma*S;
end

== matlab function MiniHelicopterControl/Q/Subsystem2/Skew_fcn2 ==
  data: vec input; S output
function S = fcn(vec)
v = vec;
vx = v(1);
vy = v(2);
vz = v(3);

S = [ ...
    0, -vz, vy; ...
    vz, 0, -vx; ...
    -vy, vx, 0 ...
    ];
end

== matlab function MiniHelicopterControl/Q/MATLAB Function13 ==
  data: Qc input size=[3 1]; Qc_ddot output size=[3 1]; xi input; wn input; z1 input; dz1 input
function Qc_ddot= fcn(Qc,xi,wn,z1,dz1)
ddz1 = -2*xi*wn*dz1-wn*(z1-Qc);
Qc_ddot = ddz1;
end

== matlab function MiniHelicopterControl/Dynamic/Subsystem/Skew_fcn ==
  data: vec input; S output
function S = fcn(vec)
v = vec;
vx = v(1);
vy = v(2);
vz = v(3);

S = [ ...
    0, -vz, vy; ...
    vz, 0, -vx; ...
    -vy, vx, 0 ...
    ];
end

== matlab function MiniHelicopterControl/Dynamic/Subsystem/G_matConstraction ==
  data: q input; sigma input; G output; S input
function G = fcn(q, sigma, S)
G = 0.5.*[-1.*q';...
    sigma.*eye(3) + S];
end

== matlab function MiniHelicopterControl/Force&Torque/f_deltaConstraction ==
  data: T_m input; f_delta output; as input; bs input; T_t input
function f_delta = fcn(T_m, as, bs, T_t)
f_delta = [T_m*sin(as);
    -T_m*sin(bs)+T_t;
    T_m*(cos(as)*cos(bs)-1)];
end

== matlab function MiniHelicopterControl/Force&Torque/fConstraction ==
  data: T_m input; f output; f_delta input
function f = fcn(T_m, f_delta)
f = T_m.*[0; 0; 1] + f_delta;
end

== matlab function MiniHelicopterControl/Force&Torque/tauConstration ==
  data: tau_gamma input; tau output; delta_tau input
function tau = fcn(tau_gamma, delta_tau)
tau = tau_gamma + delta_tau;
end

== matlab function MiniHelicopterControl/Force&Torque/delta_tauConstration ==
  data: tau_m input; delta_tau output; as input; bs input; hm input; lm input; tau_t input; T_m input
function delta_tau = fcn(tau_m, as, bs, hm, lm, tau_t, T_m)
delta_tau = [tau_m*(sin(as)-as) + T_m*hm*(sin(bs)-bs);
    tau_t - tau_m*(sin(bs)-bs) + T_m*hm*(sin(as)-as);
    tau_m*(cos(as)*cos(bs)-1) - T_m*lm*(sin(bs)-bs)];
end
